simulink model "state_observer_controller"  (R2019b)
settings: Solver=VariableStepAuto  StartTime=0.0  StopTime=30  RelTol=1e-6
values from neighbouring files (symbols this model uses):
  A = [0 1; -2 3]    [Kalman_FSFB.m]    (also in LQR_MSD.m = [0      1)
  B = [0 1]'    [Kalman_FSFB.m]    (also in LQR_MSD.m = [0)
  C = [1 1]    [Kalman_FSFB.m]    (also in LQR_MSD.m = eye(2))
  K = lqr(A,B1,eye(2),0.25)    [Kalman_FSFB.m]
  L = P*C'/(D*D')    [Kalman_FSFB.m]
settings Model: Creator=bala4krish  LastModifiedBy=bala4krish

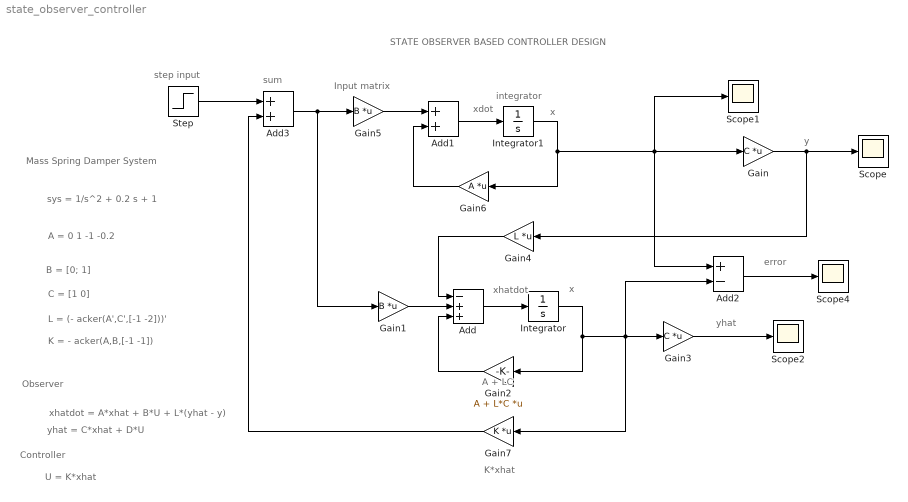
== system state_observer_controller ==
  note: error
  note: U = K*xhat
  note: Controller
  note: yhat = C*xhat + D*U
  note: xhatdot = A*xhat + B*U + L*(yhat - y)
  note: Observer
  note: Mass Spring Damper System
  note: K*xhat
  note: A + LC
  note: sys = 1/s^2 + 0.2 s + 1
  note: K = - acker(A,B,[-1 -1])
  note: L = (- acker(A',C',[-1 -2]))'
  note: C = [1 0]
  note: B = [0; 1]
  note: A =   0     1
      | 	-1   -0.2
  note: yhat
  note: y
  note: x
  note: xhatdot
  note: x
  note: xdot
  note: integrator
  note: Input matrix
  note: sum
  note: step input
  note: STATE OBSERVER BASED CONTROLLER DESIGN
  Add : Sum  Inputs=-++
  Add1 : Sum
  Add2 : Sum  Inputs=+-
  Add3 : Sum
  Gain : Gain  Gain=C  Multiplication=Matrix(K*u)
  Gain1 : Gain  Gain=B  Multiplication=Matrix(K*u)
  Gain2 : Gain  Gain=A + L*C  Multiplication=Matrix(K*u)
  Gain3 : Gain  Gain=C  Multiplication=Matrix(K*u)
  Gain4 : Gain  Gain=L  Multiplication=Matrix(K*u)
  Gain5 : Gain  Gain=B  Multiplication=Matrix(K*u)
  Gain6 : Gain  Gain=A  Multiplication=Matrix(K*u)
  Gain7 : Gain  Gain=K  Multiplication=Matrix(K*u)
  Integrator : Integrator
  Integrator1 : Integrator
  Scope{,1..2,4} (4 alike) : Scope
  Step : Step  Time=0  SampleTime=0
  wires:
  Integrator/1 -> Gain7/1, Add2/2, Gain3/1, Gain2/1
  Gain3/1 -> Scope2/1
  Gain5/1 -> Add1/1
  Gain1/1 -> Add/2
  Gain4/1 -> Add/1
  Gain2/1 -> Add/3
  Integrator1/1 -> Scope1/1, Add2/1, Gain/1, Gain6/1
  Add/1 -> Integrator/1
  Gain/1 -> Scope/1, Gain4/1
  Gain6/1 -> Add1/2
  Add1/1 -> Integrator1/1
  Add2/1 -> Scope4/1
  Add3/1 -> Gain1/1, Gain5/1
  Step/1 -> Add3/1
  Gain7/1 -> Add3/2
